simulink model "ducted_fan_tailsitter"  (R2022b)
settings: Solver=VariableStepAuto  StartTime=0.0  StopTime=100.0  FixedStep=0.2  RelTol=1e-3
InitFcn:
  | parameters
undefined symbols (not defined in the file or in its folder): pa, ToDeg, ToRad
settings Model: Creator=Administrator  LastModifiedBy=HQ03
settings SolverCC: AlgebraicLoopSolver=TrustRegion
settings DebuggingCC: UnconnectedInputMsg=warning  UnconnectedOutputMsg=warning  UnconnectedLineMsg=warning  SFMachineParentedDataDiag=warning
settings ModelReferenceCC: EnableRefExpFcnMdlSchedulingChecks=on

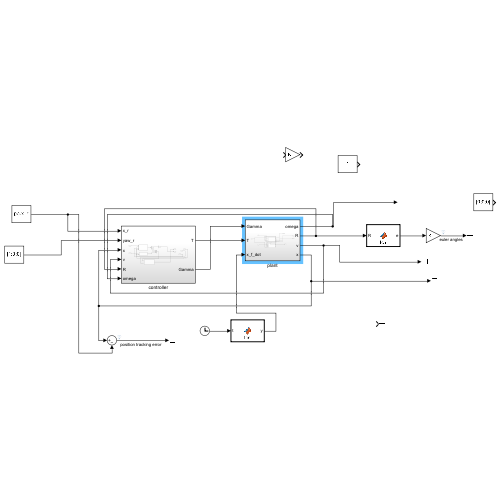
[thumbnail: Simulink's stored preview of the top-level diagram]
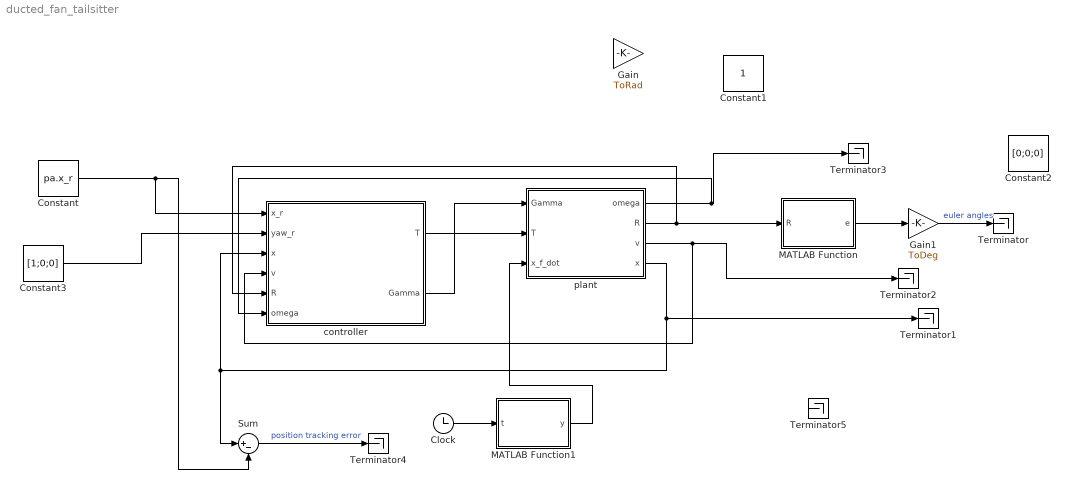
== system ducted_fan_tailsitter ==
  Clock : Clock
  Constant : Constant  Value=pa.x_r
  Constant1 : Constant
  Constant2 : Constant  Value=[0;0;0]
  Constant3 : Constant  Value=[1;0;0]
  Gain : Gain  Gain=ToRad
  Gain1 : Gain  Gain=ToDeg
  MATLAB Function : MATLAB Function  TreatAsAtomicUnit=on
  MATLAB Function1 : MATLAB Function  TreatAsAtomicUnit=on
  Sum : Sum  Inputs=|+-
  Terminator{,1..5} (6 alike) : Terminator
  controller : Subsystem
  plant : Subsystem
  wires:
  MATLAB Function/1(e) -> Gain1/1
  Gain1/1 -> Terminator/1  "euler angles"
  MATLAB Function1/1(y) -> plant/3(x_f_dot)
  plant/1(omega) -> controller/6(omega), Terminator3/1
  plant/3(v) -> controller/4(v), Terminator2/1
  plant/4(x) -> Sum/1, controller/3(x), Terminator1/1
  plant/2(R) -> controller/5(R), MATLAB Function/1(R)
  Constant/1 -> Sum/2, controller/1(x_r)
  Constant3/1 -> controller/2(yaw_r)
  controller/2(Gamma) -> plant/1(Gamma)
  controller/1(T) -> plant/2(T)
  Sum/1 -> Terminator4/1  "position tracking error"
  Clock/1 -> MATLAB Function1/1(t)

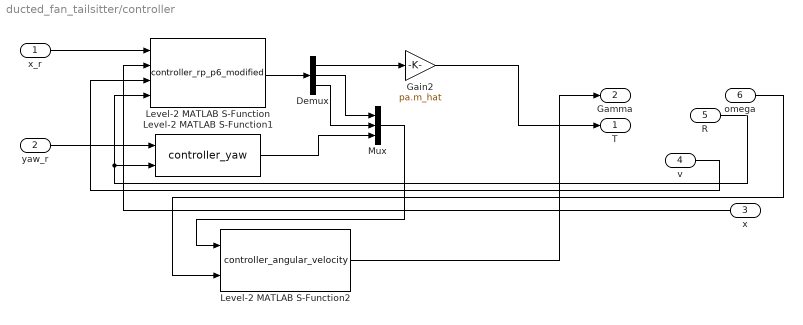
== system ducted_fan_tailsitter/controller ==
  x_r : Inport
  yaw_r : Inport  Port=2
  x : Inport  Port=3
  v : Inport  Port=4
  R : Inport  Port=5
  omega : Inport  Port=6
  Demux : Demux  Outputs=3
  Gain2 : Gain  Gain=pa.m_hat
  Level-2 MATLAB S-Function : M-S-Function  FunctionName=controller_rp_p6_modified  Parameters=pa
  Level-2 MATLAB S-Function1 : M-S-Function  FunctionName=controller_yaw  Parameters=pa
  Level-2 MATLAB S-Function2 : M-S-Function  FunctionName=controller_angular_velocity  Parameters=pa
  Mux : Mux  Inputs=3
  T : Outport
  Gamma : Outport  Port=2
  wires:
  Demux/2 -> Mux/1
  Mux/1 -> Level-2 MATLAB S-Function2/1
  Demux/1 -> Gain2/1
  R/1 -> Level-2 MATLAB S-Function1/2, Level-2 MATLAB S-Function/4
  Level-2 MATLAB S-Function/1 -> Demux/1
  Level-2 MATLAB S-Function2/1 -> Gamma/1
  Gain2/1 -> T/1
  v/1 -> Level-2 MATLAB S-Function/3
  Demux/3 -> Mux/2
  Level-2 MATLAB S-Function1/1 -> Mux/3
  omega/1 -> Level-2 MATLAB S-Function2/2
  x/1 -> Level-2 MATLAB S-Function/2
  x_r/1 -> Level-2 MATLAB S-Function/1
  yaw_r/1 -> Level-2 MATLAB S-Function1/1

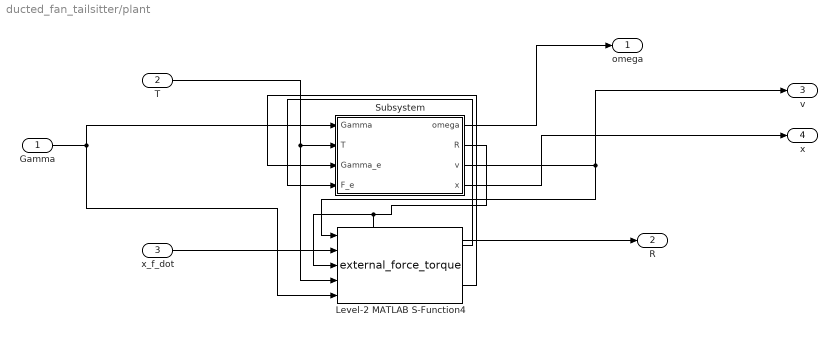
== system ducted_fan_tailsitter/plant ==
  Gamma : Inport
  T : Inport  Port=2
  x_f_dot : Inport  Port=3
  Level-2 MATLAB S-Function4 : M-S-Function  FunctionName=external_force_torque  Parameters=pa
  Subsystem : Subsystem
  omega : Outport
  R : Outport  Port=2
  v : Outport  Port=3
  x : Outport  Port=4
  wires:
  Subsystem/1(omega) -> omega/1
  Level-2 MATLAB S-Function4/2 -> Subsystem/3(Gamma_e)
  x_f_dot/1 -> Level-2 MATLAB S-Function4/2
  Level-2 MATLAB S-Function4/1 -> Subsystem/4(F_e)
  Subsystem/2(R) -> R/1, Level-2 MATLAB S-Function4/3
  T/1 -> Level-2 MATLAB S-Function4/4, Subsystem/2(T)
  Subsystem/3(v) -> v/1, Level-2 MATLAB S-Function4/1
  Subsystem/4(x) -> x/1
  Gamma/1 -> Level-2 MATLAB S-Function4/5, Subsystem/1(Gamma)

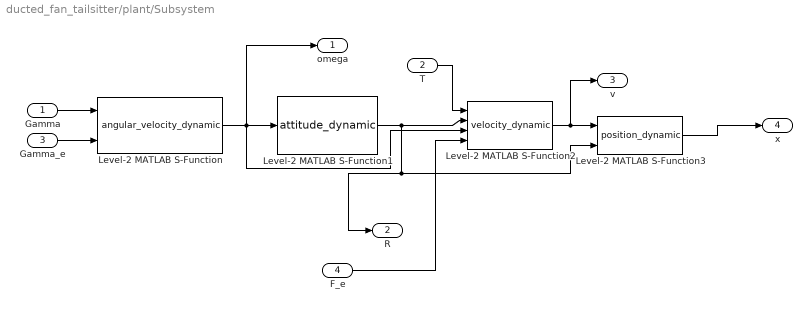
== system ducted_fan_tailsitter/plant/Subsystem ==
  Gamma : Inport
  T : Inport  Port=2
  Gamma_e : Inport  Port=3
  F_e : Inport  Port=4
  Level-2 MATLAB S-Function : M-S-Function  FunctionName=angular_velocity_dynamic  Parameters=pa
  Level-2 MATLAB S-Function1 : M-S-Function  FunctionName=attitude_dynamic
  Level-2 MATLAB S-Function2 : M-S-Function  FunctionName=velocity_dynamic  Parameters=pa
  Level-2 MATLAB S-Function3 : M-S-Function  FunctionName=position_dynamic  Parameters=pa
  omega : Outport
  R : Outport  Port=2
  v : Outport  Port=3
  x : Outport  Port=4
  wires:
  F_e/1 -> Level-2 MATLAB S-Function2/4
  Level-2 MATLAB S-Function/1 -> omega/1, Level-2 MATLAB S-Function2/3, Level-2 MATLAB S-Function1/1
  Level-2 MATLAB S-Function2/1 -> v/1, Level-2 MATLAB S-Function3/1
  Level-2 MATLAB S-Function1/1 -> Level-2 MATLAB S-Function2/2, R/1, Level-2 MATLAB S-Function3/2
  Gamma_e/1 -> Level-2 MATLAB S-Function/2
  Level-2 MATLAB S-Function3/1 -> x/1
  T/1 -> Level-2 MATLAB S-Function2/1
  Gamma/1 -> Level-2 MATLAB S-Function/1

== matlab function ducted_fan_tailsitter/MATLAB Function ==
  data: R input; e output
function e = fcn(R)

e = zeros(3,1);
e(1) = atan2(R(3,2),R(3,3));
e(2) = -asin(R(3,1));
e(3) = atan2(R(2,1),R(1,1));

== matlab function ducted_fan_tailsitter/MATLAB Function1 ==
  data: t input; y output
function y = fcn(t)

if t<=30
    x_f_dot = [0;0;0];
elseif (t>30) && (t<=70)
    x_f_dot = [4;0;0];
else
    x_f_dot = [8;0;0];
end

y = x_f_dot;
